simulink model "sandbox_application"  (R2020b)
settings: Solver=FixedStepAuto  StartTime=0.0  StopTime=0.5  FixedStep=250e-6  RelTol=1e-3  EnableMultiTasking=on
PreLoadFcn:
  | init
libraries: sandbox_lib x9, simulink x4, slpidlib x1
settings Model: Creator=CHOLSCH3  LastModifiedBy=INCHNR2
settings OptimizationCC: DefaultParameterBehavior=Inlined  EnhancedBackFolding=on  PassReuseOutputArgsThreshold=0  MaxStackSize=1024  OptimizeBlockOrder=speed  DifferentSizesBufferReuse=on  OptimizationCustomize=off
settings DebuggingCC: ParameterTunabilityLossMsg=error
settings HardwareCC: ProdBitPerLong=64  ProdLargestAtomicInteger=LongLong  ProdLargestAtomicFloat=Double  ProdLongLongMode=on  ProdHWDeviceType=ARM Compatible->ARM 64-bit (LP64)
settings SFSimCC: MATLABDynamicMemAlloc=off  SimTargetLang=C++
settings SFSimCC: SimCustomSourceCode=|
  | const uint32_t num_entries = 256;
  | static std::uint32_t storage[num_entries][num_entries] = {};
  | 
  | bool write_parameter_float(std::uint32_t group, std::uint32_t index, float value)
  | {
  |     if(group>=num_entries || index >= num_entries)
  |         return false;
  | 
  |     *(float *)&storage[group][index] = value;
  |     return true;
  | }
  | float read_parameter_float(std::uint32_t group, std::uint32_t index)
  | {
  |     if(group>=num_entries || index >= num_entries)
  |         return 0.0f;
  | 
  |     return *(float *)&storage[group][index];
  | }
  | bool write_parameter_int32(uint32_t group, uint32_t index, int32_t value)
  | {
  |     if(group>=num_entries || index >= num_entries)
  |         return false;
  | 
  |     *(int32_t *)&storage[group][index] = value;
  |     return true;
  | }
  | int32_t read_parameter_int32(uint32_t group, uint32_t index)
  | {
  |     if(group>=num_entries || index >= num_entries)
  |         return 0;
  | 
  |     return *(int32_t *)&storage[group][index];
  | }
settings SFSimCC: SimCustomHeaderCode=|
  | #include <cstdint>
  | bool write_parameter_float(std::uint32_t group, std::uint32_t index, float value);
  | float read_parameter_float(std::uint32_t group, std::uint32_t index);
  | bool write_parameter_int32(uint32_t group, uint32_t index, int32_t value);
  | int32_t read_parameter_int32(uint32_t group, uint32_t index);
settings RTWCC: GenCodeOnly=on  PackageName=test.zip  GenerateReport=on  RTWVerbose=off  CustomHeaderCode="#include \"syscalls.h\""  Toolchain=MinGW64 | gmake (64-bit Windows)  LaunchReport=on  TargetLang=C++
settings CodeAppCC: ForceParamTrailComments=on  OperatorAnnotations=on
settings GRTTargetCC: TargetLangStandard=C++03 (ISO)  MatFileLogging=off

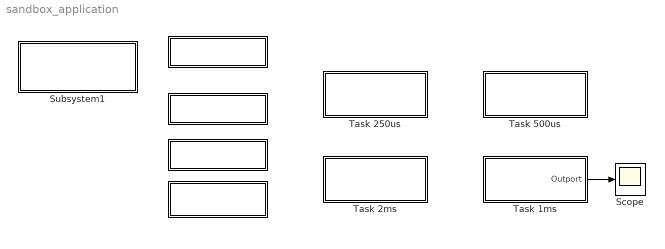
== system sandbox_application ==
  " " : Subsystem
      settings: AttributesFormatString=%<BlockChoice>  OpenFcn=build('UCU');
      mask Display: disp('Build for UCU');
  "  " : Subsystem
      settings: OpenFcn=build('PC_32bit');
      mask Display: disp('Build for PC 32bit');
  "   " : Subsystem
      settings: OpenFcn=build('PC 64bit');
      mask Display: disp('Build for PC 64bit');
  "    " : Subsystem
      settings: OpenFcn=build('all');
      mask Display: disp('Build all');
  Scope : Scope
  Subsystem1 : Subsystem
      settings: OpenFcn="build(\"all\")"  MinAlgLoopOccurrences=on
      mask Display: disp("Build for All")
  Task 1ms : Subsystem  TreatAsAtomicUnit=on  SystemSampleTime=1e-3
  Task 250us : Subsystem  LoadFcn=init  TreatAsAtomicUnit=on  SystemSampleTime=250e-6
  Task 2ms : Subsystem  TreatAsAtomicUnit=on  SystemSampleTime=2e-3
  Task 500us : Subsystem  TreatAsAtomicUnit=on  SystemSampleTime=500e-6
  wires:
  Task 1ms/1(Outport) -> Scope/1

== system sandbox_application/  ==

== system sandbox_application/   ==

== system sandbox_application/    ==

== system sandbox_application/     ==

== system sandbox_application/Subsystem1 ==

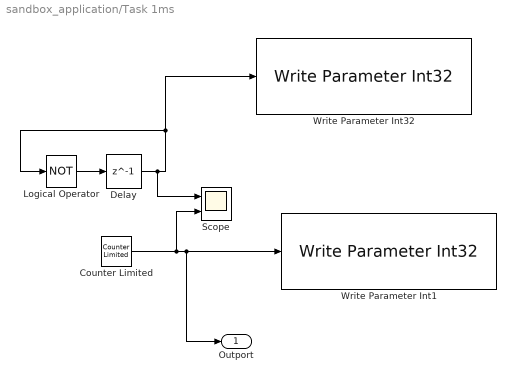
== system sandbox_application/Task 1ms ==
  Counter Limited : simulink/Sources/Counter Limited  uplimit=9  tsamp=-1
  Delay : Delay  DelayLength=1
  Logical Operator : Logic  Operator=NOT  AllPortsSameDT=off  OutDataTypeStr=boolean
  Scope : Scope  NumInputPorts=2
  Write Parameter Int1 : sandbox_lib/Write Parameter Int32  parameter_group=47  parameter_index=15
  Write Parameter Int32 : sandbox_lib/Write Parameter Int32  parameter_group=47  parameter_index=14
  Outport : Outport
  wires:
  Delay/1 -> Scope/1, Write Parameter Int32/1, Logical Operator/1
  Logical Operator/1 -> Delay/1
  Counter Limited/1 -> Scope/2, Outport/1, Write Parameter Int1/1

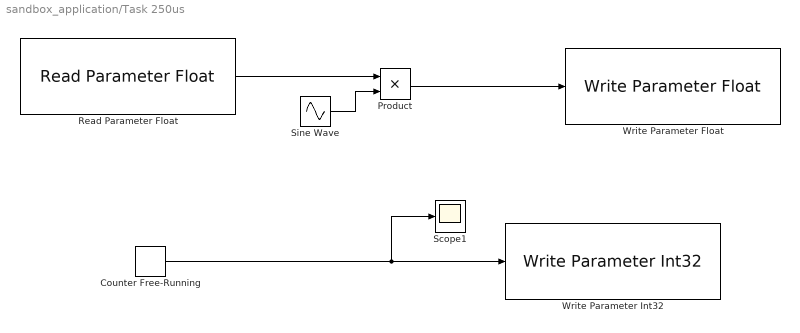
== system sandbox_application/Task 250us ==
  Counter Free-Running : simulink/Sources/Counter Free-Running  NumBits=4  tsamp=-1
  Product : Product  OutDataTypeStr=fixdt(1,16,10)
  Read Parameter Float : sandbox_lib/Read Parameter Float  parameter_group=47  parameter_index=05
  Scope1 : Scope
  Sine Wave : Sin  Frequency=2*pi*10  SampleTime=250e-6
  Write Parameter Float : sandbox_lib/Write Parameter Float  parameter_group=47  parameter_index=02
  Write Parameter Int32 : sandbox_lib/Write Parameter Int32  parameter_group=47  parameter_index=11
  wires:
  Product/1 -> Write Parameter Float/1
  Sine Wave/1 -> Product/2
  Read Parameter Float/1 -> Product/1
  Counter Free-Running/1 -> Scope1/1, Write Parameter Int32/1

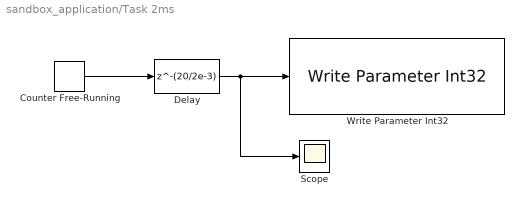
== system sandbox_application/Task 2ms ==
  Counter Free-Running : simulink/Sources/Counter Free-Running  NumBits=16  tsamp=-1
  Delay : Delay  DelayLength=(20/2e-3)
  Scope : Scope
  Write Parameter Int32 : sandbox_lib/Write Parameter Int32  parameter_group=47  parameter_index=13
  wires:
  Counter Free-Running/1 -> Delay/1
  Delay/1 -> Scope/1, Write Parameter Int32/1

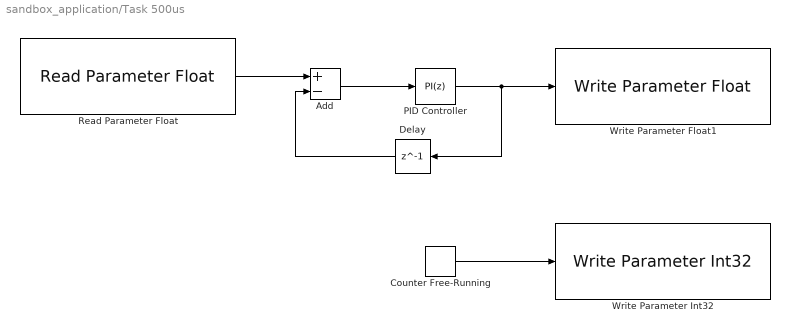
== system sandbox_application/Task 500us ==
  Add : Sum  Inputs=+-
  Counter Free-Running : simulink/Sources/Counter Free-Running  NumBits=32  tsamp=-1
  Delay : Delay  DelayLength=1
  PID Controller : slpidlib/PID Controller  Controller=PI  Form=Parallel  TimeDomain=Discrete-time  UseExternalTs=off  SampleTime=-1  IntegratorMethod=Forward Euler  FilterMethod=Forward Euler  ControllerParametersSource=internal  P=0.1  I=10  D=0  UseFilter=on  N=100  TunerSelectOption=Transfer Function Based (PID Tuner App)  InitialConditionSource=internal  InitialConditionForIntegrator=0  InitialConditionForFilter=0  DifferentiatorICPrevScaledInput=0  ExternalReset=none  TrackingMode=off  Kt=1  LimitOutput=off  SatLimitsSource=internal  UpperSaturationLimit=inf  LowerSaturationLimit=-inf  LinearizeAsGain=on  AntiWindupMode=none  Kb=1  POutMin=[]  POutMax=[]  IOutMin=[]  IOutMax=[]  DOutMin=[]  DOutMax=[]  NOutMin=[]  NOutMax=[]  SumOutMin=[]  SumOutMax=[]  SaturationOutMin=[]  SaturationOutMax=[]  PParamMin=[]  PParamMax=[]  IParamMin=[]  IParamMax=[]  DParamMin=[]  DParamMax=[]  NParamMin=[]  NParamMax=[]  KbParamMin=[]  KbParamMax=[]  KtParamMin=[]  KtParamMax=[]  KbOutMin=[]  KbOutMax=[]  KtOutMin=[]  KtOutMax=[]  IntegratorOutMin=[]  IntegratorOutMax=[]  FilterOutMin=[]  FilterOutMax=[]  SumI1OutMin=[]  SumI1OutMax=[]  SumI2OutMin=[]  SumI2OutMax=[]  SumI3OutMin=[]  SumI3OutMax=[]  SumI4OutMin=[]  SumI4OutMax=[]  SumDOutMin=[]  SumDOutMax=[]  DifferentiatorOutMin=[]  DifferentiatorOutMax=[]  FilterDiffOutCoefMin=[]  FilterDiffOutCoefMax=[]  ReciprocalOutMin=[]  ReciprocalOutMax=[]  SumDenOutMin=[]  SumDenOutMax=[]  SumNumOutMin=[]  SumNumOutMax=[]  DivideOutMin=[]  DivideOutMax=[]  UdiffTsProdOutMin=[]  UdiffTsProdOutMax=[]  NTsProdOutMin=[]  NTsProdOutMax=[]  UintegralTsProdOutMin=[]  UintegralTsProdOutMax=[]  UngainTsProdOutMin=[]  UngainTsProdOutMax=[]  IntegratorContinuousStateAttributes=''  IntegratorStateMustResolveToSignalObject=off  IntegratorRTWStateStorageClass=Auto  FilterContinuousStateAttributes=''  FilterStateMustResolveToSignalObject=off  FilterRTWStateStorageClass=Auto  ParallelPVariant=InternalParameters  IdealPVariant=Disabled  IVariant=InternalParameters  DVariant=Disabled  IntegratorVariant=Discrete  SatVariant=Disabled  AWVariant=Passthrough  PCopyVariant=Disabled  TRVariant=Disabled  FdbkBlocksVariant=Forward  IdealPFdbkVariant=Disabled  SatFdbkVariant=Disabled  DerivativeFilterVariant=Disabled  NVariant=Disabled  NCopyVariant=Disabled_SignalSpec  FilterICVariant=Disabled  IntegratorICVariant=InternalICs  ExternalResetVariant=Disabled  TRSumVariant=Passthrough  SumFdbkVariant=Disabled  SumVariant=Sum_PI  TsampFilterVariant=InternalTs  TsampNgainVariant=Passthrough  TsampIntegralVariant=Passthrough  ExternalSaturationOutDataTypeStr=Inherit: Same as second input
  Read Parameter Float : sandbox_lib/Read Parameter Float  parameter_group=47  parameter_index=01
  Write Parameter Float1 : sandbox_lib/Write Parameter Float  parameter_group=47  parameter_index=03
  Write Parameter Int32 : sandbox_lib/Write Parameter Int32  parameter_group=47  parameter_index=12
  wires:
  Counter Free-Running/1 -> Write Parameter Int32/1
  PID Controller/1 -> Write Parameter Float1/1, Delay/1
  Delay/1 -> Add/2
  Read Parameter Float/1 -> Add/1
  Add/1 -> PID Controller/1
